simulink model "VIPL4sStEnCtrl"  (R2018b)
settings: Solver=FixedStepDiscrete  StartTime=0.0  StopTime=10.0  FixedStep=0.01  RelTol=1e-3
undefined symbols (not defined in the file or in its folder): data, KeSMSw4SSecRwLtStLgrstUpwdDnwdOpenPos1_Val, SecRwLtStBkReclnEn_Clear, SecRwLtStBkReclnEn_Set, SecRwLtStFtrstEn_Clear, SecRwLtStFtrstEn_Set, SecRwLtStFwdBkwdEn_Clear, SecRwLtStFwdBkwdEn_Set, SecRwLtStHdrstFwdBkwdEn_Clear, SecRwLtStHdrstFwdBkwdEn_Set, SecRwLtStHdrstUpwdDnwdEn_Clear, SecRwLtStHdrstUpwdDnwdEn_Set, SecRwLtStLgrstInwdOtwdEn_Clear, SecRwLtStLgrstInwdOtwdEn_Set, SecRwLtStLgrstUpwdDnwdEn_Clear, SecRwLtStLgrstUpwdDnwdEn_Set
libraries: simulink x16
settings Model: ModifiedHistory="2023.11.16  V2.3.0 Issue 566045 全躺，vip，腿托打开增加前后位置"  Creator=sn2xws  LastModifiedBy=sn2xws
settings DataIOCC: SaveFormat=StructureWithTime
settings OptimizationCC: DefaultParameterBehavior=Inlined  EnhancedBackFolding=on  PassReuseOutputArgsAs=Individual arguments  ZeroExternalMemoryAtStartup=off  ZeroInternalMemoryAtStartup=off  OptimizeBlockOrder=speed  DifferentSizesBufferReuse=on  OptimizationCustomize=off
settings DebuggingCC: ParameterTunabilityLossMsg=error
settings SFSimCC: MATLABDynamicMemAlloc=off
settings RTWCC: SystemTargetFile=autosar.tlc  GenCodeOnly=on  TemplateMakefile=ert_default_tmf  Description=AUTOSAR  GenerateReport=on  IncludeHyperlinkInReport=on  LaunchReport=on  GenerateTraceInfo=on  GenerateTraceReport=on  GenerateTraceReportSl=on  GenerateTraceReportSf=on  GenerateTraceReportEml=on  GenerateCodeMetricsReport=on
settings CodeAppCC: ForceParamTrailComments=on  IgnoreCustomStorageClasses=off  OperatorAnnotations=on  SimulinkDataObjDesc=on  SFDataObjDesc=on  InsertBlockDesc=on
settings STFCustomTargetCC: TargetLangStandard=C99 (ISO)  MultiwordLength=256  ParMdlRefBuildCompliant=on  CompOptLevelCompliant=on  IncludeMdlTerminateFcn=off  CombineOutputUpdateFcns=on  SuppressErrorStatus=on  ERTCustomFileBanners=on  SupportNonFinite=off  SupportComplex=off  SupportContinuousTime=off  SupportNonInlinedSFcns=off  RemoveResetFunc=on  MATLABClassNameForMDSCustomization=Simulink.SoftwareTarget.ERTCustomization  AutosarCompliant=on  UseToolchainInfoCompliant=on  LookupTableObjectStructAxisOrder=2,1,3,4,...  LUTObjectStructOrderEvenSpacing=Size,Table,Breakpoints  SystemTargetFile=autosar.tlc
settings ERTTargetCC: TargetLangStandard=C99 (ISO)  ConcurrentExecutionCompliant=off  IncludeMdlTerminateFcn=off  SuppressErrorStatus=on  SupportNonFinite=off  SupportComplex=off  ModelStepFunctionPrototypeControlCompliant=off  CPPClassGenCompliant=off  AutosarCompliant=on  LookupTableObjectStructAxisOrder=2,1,3,4,...  LUTObjectStructOrderEvenSpacing=Size,Table,Breakpoints  InlinedParameterPlacement=NonHierarchical  ERTCustomFileTemplate=example_file_process.tlc  ERTFilePackagingFormat=Compact

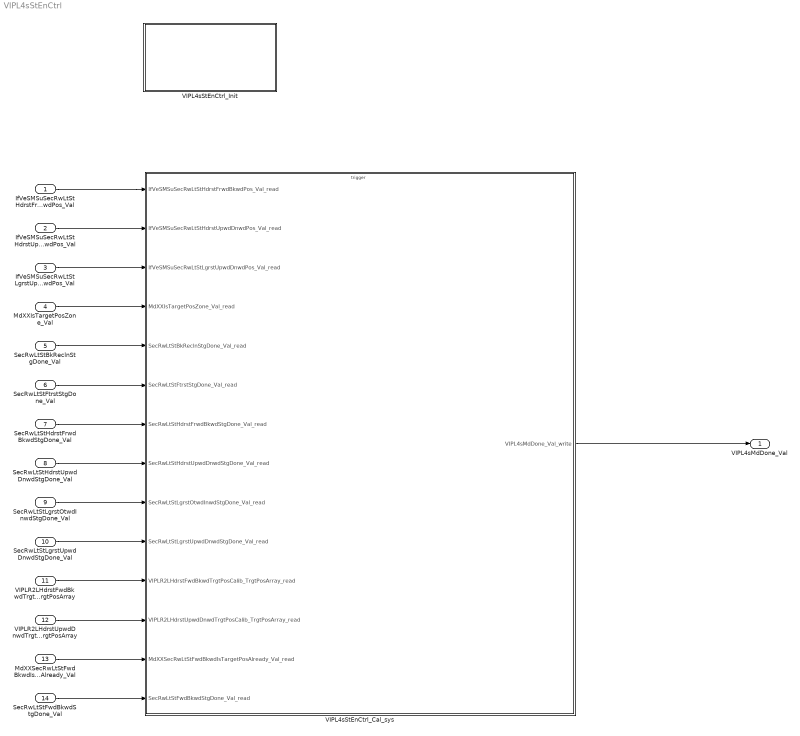
== system VIPL4sStEnCtrl ==
  IfVeSMSuSecRwLtStHdrstFrwdBkwdPos_Val : Inport  OutDataTypeStr=uint16  PortDimensions=1
  IfVeSMSuSecRwLtStHdrstUpwdDnwdPos_Val : Inport  Port=2  OutDataTypeStr=uint16  PortDimensions=1
  IfVeSMSuSecRwLtStLgrstUpwdDnwdPos_Val : Inport  Port=3  OutDataTypeStr=uint16  PortDimensions=1
  MdXXIsTargetPosZone_Val : Inport  Port=4  OutDataTypeStr=uint32  PortDimensions=1
  SecRwLtStBkReclnStgDone_Val : Inport  Port=5  OutDataTypeStr=boolean  PortDimensions=1
  SecRwLtStFtrstStgDone_Val : Inport  Port=6  OutDataTypeStr=boolean  PortDimensions=1
  SecRwLtStHdrstFrwdBkwdStgDone_Val : Inport  Port=7  OutDataTypeStr=boolean  PortDimensions=1
  SecRwLtStHdrstUpwdDnwdStgDone_Val : Inport  Port=8  OutDataTypeStr=boolean  PortDimensions=1
  SecRwLtStLgrstOtwdInwdStgDone_Val : Inport  Port=9  OutDataTypeStr=boolean  PortDimensions=1
  SecRwLtStLgrstUpwdDnwdStgDone_Val : Inport  Port=10  OutDataTypeStr=boolean  PortDimensions=1
  VIPLR2LHdrstFwdBkwdTrgtPosCalib_TrgtPosArray : Inport  Description=|  Port=11  OutDataTypeStr=uint16  PortDimensions=3
      | 0:Pos
      | 1:Max
      | 2:Min
  VIPLR2LHdrstUpwdDnwdTrgtPosCalib_TrgtPosArray : Inport  Description=|  Port=12  OutDataTypeStr=uint16  PortDimensions=3
      | 0:Pos
      | 1:Max
      | 2:Min
  MdXXSecRwLtStFwdBkwdIsTargetPosAlready_Val : Inport  Port=13  OutDataTypeStr=uint32  PortDimensions=1
  SecRwLtStFwdBkwdStgDone_Val : Inport  Port=14  OutDataTypeStr=boolean  PortDimensions=1
  VIPL4sStEnCtrl_Cal_sys : Subsystem
  VIPL4sStEnCtrl_Init : Subsystem
  VIPL4sMdDone_Val : Outport  OutDataTypeStr=uint8  PortDimensions=1
  wires:
  IfVeSMSuSecRwLtStHdrstFrwdBkwdPos_Val/1 -> VIPL4sStEnCtrl_Cal_sys/1(IfVeSMSuSecRwLtStHdrstFrwdBkwdPos_Val_read)
  IfVeSMSuSecRwLtStHdrstUpwdDnwdPos_Val/1 -> VIPL4sStEnCtrl_Cal_sys/2(IfVeSMSuSecRwLtStHdrstUpwdDnwdPos_Val_read)
  IfVeSMSuSecRwLtStLgrstUpwdDnwdPos_Val/1 -> VIPL4sStEnCtrl_Cal_sys/3(IfVeSMSuSecRwLtStLgrstUpwdDnwdPos_Val_read)
  MdXXIsTargetPosZone_Val/1 -> VIPL4sStEnCtrl_Cal_sys/4(MdXXIsTargetPosZone_Val_read)
  SecRwLtStBkReclnStgDone_Val/1 -> VIPL4sStEnCtrl_Cal_sys/5(SecRwLtStBkReclnStgDone_Val_read)
  SecRwLtStFtrstStgDone_Val/1 -> VIPL4sStEnCtrl_Cal_sys/6(SecRwLtStFtrstStgDone_Val_read)
  SecRwLtStHdrstFrwdBkwdStgDone_Val/1 -> VIPL4sStEnCtrl_Cal_sys/7(SecRwLtStHdrstFrwdBkwdStgDone_Val_read)
  SecRwLtStHdrstUpwdDnwdStgDone_Val/1 -> VIPL4sStEnCtrl_Cal_sys/8(SecRwLtStHdrstUpwdDnwdStgDone_Val_read)
  SecRwLtStLgrstOtwdInwdStgDone_Val/1 -> VIPL4sStEnCtrl_Cal_sys/9(SecRwLtStLgrstOtwdInwdStgDone_Val_read)
  SecRwLtStLgrstUpwdDnwdStgDone_Val/1 -> VIPL4sStEnCtrl_Cal_sys/10(SecRwLtStLgrstUpwdDnwdStgDone_Val_read)
  VIPLR2LHdrstFwdBkwdTrgtPosCalib_TrgtPosArray/1 -> VIPL4sStEnCtrl_Cal_sys/11(VIPLR2LHdrstFwdBkwdTrgtPosCalib_TrgtPosArray_read)
  VIPLR2LHdrstUpwdDnwdTrgtPosCalib_TrgtPosArray/1 -> VIPL4sStEnCtrl_Cal_sys/12(VIPLR2LHdrstUpwdDnwdTrgtPosCalib_TrgtPosArray_read)
  VIPL4sStEnCtrl_Cal_sys/1(VIPL4sMdDone_Val_write) -> VIPL4sMdDone_Val/1
  MdXXSecRwLtStFwdBkwdIsTargetPosAlready_Val/1 -> VIPL4sStEnCtrl_Cal_sys/13(MdXXSecRwLtStFwdBkwdIsTargetPosAlready_Val_read)
  SecRwLtStFwdBkwdStgDone_Val/1 -> VIPL4sStEnCtrl_Cal_sys/14(SecRwLtStFwdBkwdStgDone_Val_read)

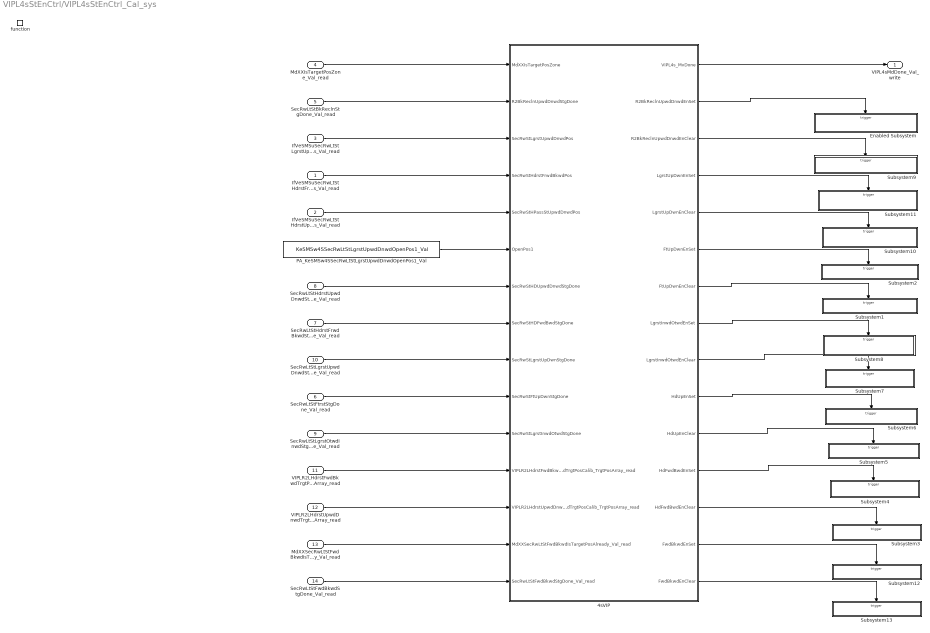
== system VIPL4sStEnCtrl/VIPL4sStEnCtrl_Cal_sys ==
  IfVeSMSuSecRwLtStHdrstFrwdBkwdPos_Val_read : Inport
  IfVeSMSuSecRwLtStHdrstUpwdDnwdPos_Val_read : Inport  Port=2
  IfVeSMSuSecRwLtStLgrstUpwdDnwdPos_Val_read : Inport  Port=3
  MdXXIsTargetPosZone_Val_read : Inport  Port=4
  SecRwLtStBkReclnStgDone_Val_read : Inport  Port=5
  SecRwLtStFtrstStgDone_Val_read : Inport  Port=6
  SecRwLtStHdrstFrwdBkwdStgDone_Val_read : Inport  Port=7
  SecRwLtStHdrstUpwdDnwdStgDone_Val_read : Inport  Port=8
  SecRwLtStLgrstOtwdInwdStgDone_Val_read : Inport  Port=9
  SecRwLtStLgrstUpwdDnwdStgDone_Val_read : Inport  Port=10
  VIPLR2LHdrstFwdBkwdTrgtPosCalib_TrgtPosArray_read : Inport  Port=11
  VIPLR2LHdrstUpwdDnwdTrgtPosCalib_TrgtPosArray_read : Inport  Port=12
  MdXXSecRwLtStFwdBkwdIsTargetPosAlready_Val_read : Inport  Port=13
  SecRwLtStFwdBkwdStgDone_Val_read : Inport  Port=14
  function : TriggerPort  TriggerType=function-call  IsSimulinkFunction=on  FunctionName=VIPL4sStEnCtrl_Cal  VariantControl=(inherit)
  4sVIP : Subsystem
  Enabled Subsystem : Subsystem  TreatAsAtomicUnit=on
  PA_KeSMSw4SSecRwLtStLgrstUpwdDnwdOpenPos1_Val : Constant  Value=KeSMSw4SSecRwLtStLgrstUpwdDnwdOpenPos1_Val
  Subsystem1 : Subsystem
  Subsystem10 : Subsystem
  Subsystem11 : Subsystem
  Subsystem12 : Subsystem
  Subsystem13 : Subsystem
  Subsystem2 : Subsystem
  Subsystem3 : Subsystem
  Subsystem4 : Subsystem
  Subsystem5 : Subsystem
  Subsystem6 : Subsystem
  Subsystem7 : Subsystem
  Subsystem8 : Subsystem
  Subsystem9 : Subsystem
  VIPL4sMdDone_Val_write : Outport
      settings: EnsureOutportIsVirtual=on
  wires:
  4sVIP/1(VIPL4s_MvDone) -> VIPL4sMdDone_Val_write/1
  PA_KeSMSw4SSecRwLtStLgrstUpwdDnwdOpenPos1_Val/1 -> 4sVIP/6(OpenPos1)
  MdXXIsTargetPosZone_Val_read/1 -> 4sVIP/1(MdXXIsTargetPosZone)
  SecRwLtStBkReclnStgDone_Val_read/1 -> 4sVIP/2(R2BkReclnUpwdDnwdStgDone)
  IfVeSMSuSecRwLtStLgrstUpwdDnwdPos_Val_read/1 -> 4sVIP/3(SecRwStLgrstUpwdDnwdPos)
  IfVeSMSuSecRwLtStHdrstFrwdBkwdPos_Val_read/1 -> 4sVIP/4(SecRwStHdrstFrwdBkwdPos)
  IfVeSMSuSecRwLtStHdrstUpwdDnwdPos_Val_read/1 -> 4sVIP/5(SecRwStHPassStUpwdDnwdPos)
  SecRwLtStFtrstStgDone_Val_read/1 -> 4sVIP/10(SecRwStFtUpDwnStgDone)
  SecRwLtStLgrstOtwdInwdStgDone_Val_read/1 -> 4sVIP/11(SecRwStLgrstInwdOtwdStgDone)
  SecRwLtStLgrstUpwdDnwdStgDone_Val_read/1 -> 4sVIP/9(SecRwStLgrstUpDwnStgDone)
  SecRwLtStHdrstFrwdBkwdStgDone_Val_read/1 -> 4sVIP/8(SecRwStHDFwdBwdStgDone)
  SecRwLtStHdrstUpwdDnwdStgDone_Val_read/1 -> 4sVIP/7(SecRwStHDUpwdDnwdStgDone)
  VIPLR2LHdrstFwdBkwdTrgtPosCalib_TrgtPosArray_read/1 -> 4sVIP/12(VIPLR2LHdrstFwdBkwdTrgtPosCalib_TrgtPosArray_read)
  VIPLR2LHdrstUpwdDnwdTrgtPosCalib_TrgtPosArray_read/1 -> 4sVIP/13(VIPLR2LHdrstUpwdDnwdTrgtPosCalib_TrgtPosArray_read)
  4sVIP/3(R2BkReclnUpwdDnwdEnClear) -> Subsystem9/Trigger
  4sVIP/12(HdFwdBwdEnSet) -> Subsystem4/Trigger
  4sVIP/6(FtUpDwnEnSet) -> Subsystem2/Trigger
  4sVIP/11(HdUpEnClear) -> Subsystem5/Trigger
  4sVIP/7(FtUpDwnEnClear) -> Subsystem1/Trigger
  4sVIP/13(HdFwdBwdEnClear) -> Subsystem3/Trigger
  4sVIP/2(R2BkReclnUpwdDnwdEnSet) -> Enabled Subsystem/Trigger
  4sVIP/10(HdUpEnSet) -> Subsystem6/Trigger
  4sVIP/4(LgrstUpDwnEnSet) -> Subsystem11/Trigger
  4sVIP/9(LgrstInwdOtwdEnClear) -> Subsystem7/Trigger
  4sVIP/8(LgrstInwdOtwdEnSet) -> Subsystem8/Trigger
  4sVIP/5(LgrstUpDwnEnClear) -> Subsystem10/Trigger
  MdXXSecRwLtStFwdBkwdIsTargetPosAlready_Val_read/1 -> 4sVIP/14(MdXXSecRwLtStFwdBkwdIsTargetPosAlready_Val_read)
  SecRwLtStFwdBkwdStgDone_Val_read/1 -> 4sVIP/15(SecRwLtStFwdBkwdStgDone_Val_read)
  4sVIP/14(FwdBkwdEnSet) -> Subsystem12/Trigger
  4sVIP/15(FwdBkwdEnClear) -> Subsystem13/Trigger

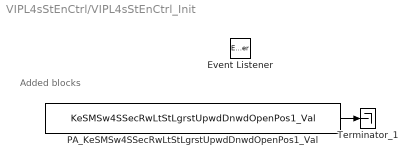
== system VIPL4sStEnCtrl/VIPL4sStEnCtrl_Init ==
  note: Added blocks
  Event Listener : EventListener  EventName=reset
  PA_KeSMSw4SSecRwLtStLgrstUpwdDnwdOpenPos1_Val : Constant  Value=KeSMSw4SSecRwLtStLgrstUpwdDnwdOpenPos1_Val
  Terminator_1 : Terminator
  wires:
  PA_KeSMSw4SSecRwLtStLgrstUpwdDnwdOpenPos1_Val/1 -> Terminator_1/1

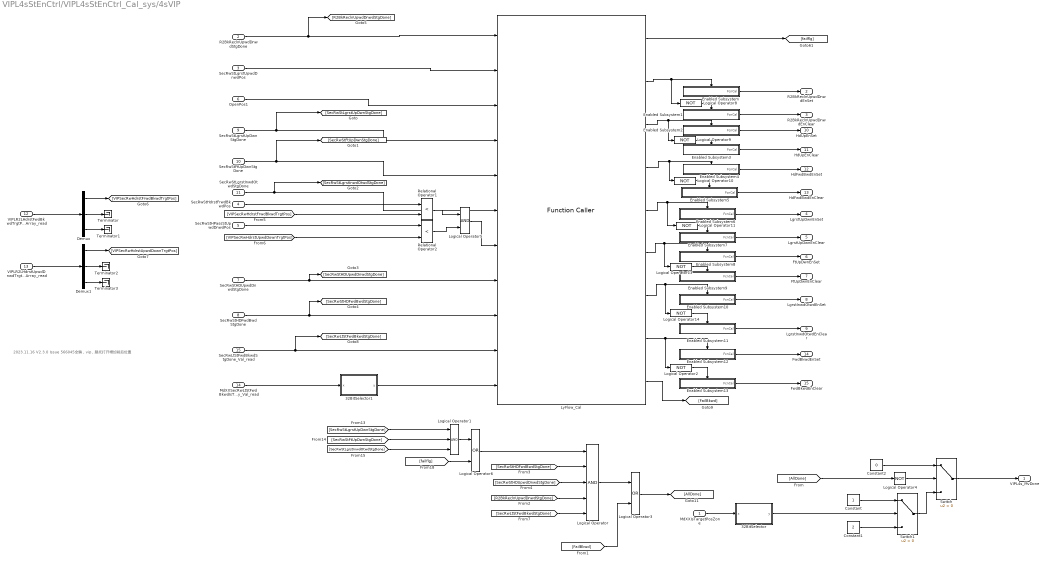
== system VIPL4sStEnCtrl/VIPL4sStEnCtrl_Cal_sys/4sVIP ==
  note: 2023.11.16 V2.3.0 Issue 566045 全躺，vip，腿托打开增加前后位置
  MdXXIsTargetPosZone : Inport
  R2BkReclnUpwdDnwdStgDone : Inport  Port=2
  SecRwStLgrstUpwdDnwdPos : Inport  Port=3
  SecRwStHdrstFrwdBkwdPos : Inport  Port=4
  SecRwStHPassStUpwdDnwdPos : Inport  Port=5
  OpenPos1 : Inport  Port=6
  SecRwStHDUpwdDnwdStgDone : Inport  Port=7
  SecRwStHDFwdBwdStgDone : Inport  Port=8
  SecRwStLgrstUpDwnStgDone : Inport  Port=9
  SecRwStFtUpDwnStgDone : Inport  Port=10
  SecRwStLgrstInwdOtwdStgDone : Inport  Port=11
  VIPLR2LHdrstFwdBkwdTrgtPosCalib_TrgtPosArray_read : Inport  Port=12
  VIPLR2LHdrstUpwdDnwdTrgtPosCalib_TrgtPosArray_read : Inport  Port=13
  MdXXSecRwLtStFwdBkwdIsTargetPosAlready_Val_read : Inport  Port=14
  SecRwLtStFwdBkwdStgDone_Val_read : Inport  Port=15
  32BitSelector : Subsystem  mask(32 Bit Selector){BitNum=9}
      mask prompts: BitNum "Select Bit Number"
      mask help: Allows selection of a particular bit (0-31) out of a packed word up to 32 bits long. Output will be true if the bit number selected via the mask parameter is equal to one.
      mask TypeOptions BitNum: 0 | 1 | 2 | 3 | 4 | 5 | 6 | 7 | 8 | 9 | 10 | 11 | 12 | 13 | 14 | 15 | 16 | 17 | 18 | 19 | 20 | 21 | 22 | 23 | 24 | 25 | 26 | 27 | 28 | 29 | 30 | 31
      mask Display:
      | text(0.5, 0.8,'BIT','horizontalAlignment','center')
      | text(0.5, 0.5,'SELECTOR','horizontalAlignment','center')
      | text(0.5, 0.2,['-- Bit ',char(get_param(gcb,'BitNum')),' --'],'horizontalAlignment','center')
  32BitSelector1 : Subsystem  mask(32 Bit Selector){BitNum=9}
      mask prompts: BitNum "Select Bit Number"
      mask help: Allows selection of a particular bit (0-31) out of a packed word up to 32 bits long. Output will be true if the bit number selected via the mask parameter is equal to one.
      mask TypeOptions BitNum: 0 | 1 | 2 | 3 | 4 | 5 | 6 | 7 | 8 | 9 | 10 | 11 | 12 | 13 | 14 | 15 | 16 | 17 | 18 | 19 | 20 | 21 | 22 | 23 | 24 | 25 | 26 | 27 | 28 | 29 | 30 | 31
      mask Display:
      | text(0.5, 0.8,'BIT','horizontalAlignment','center')
      | text(0.5, 0.5,'SELECTOR','horizontalAlignment','center')
      | text(0.5, 0.2,['-- Bit ',char(get_param(gcb,'BitNum')),' --'],'horizontalAlignment','center')
  Constant : Constant  OutDataTypeStr=uint8
  Constant1 : Constant  Value=2  OutDataTypeStr=uint8
  Constant2 : Constant  Value=0  OutDataTypeStr=uint8
  Demux : Demux  Outputs=3
  Demux1 : Demux  Outputs=3
  Enabled Subsystem : Subsystem  TreatAsAtomicUnit=on
  Enabled Subsystem1 : Subsystem  TreatAsAtomicUnit=on
  Enabled Subsystem10 : Subsystem  TreatAsAtomicUnit=on
  Enabled Subsystem11 : Subsystem  TreatAsAtomicUnit=on
  Enabled Subsystem12 : Subsystem  TreatAsAtomicUnit=on
  Enabled Subsystem13 : Subsystem  TreatAsAtomicUnit=on
  Enabled Subsystem2 : Subsystem  TreatAsAtomicUnit=on
  Enabled Subsystem3 : Subsystem  TreatAsAtomicUnit=on
  Enabled Subsystem4 : Subsystem  TreatAsAtomicUnit=on
  Enabled Subsystem5 : Subsystem  TreatAsAtomicUnit=on
  Enabled Subsystem6 : Subsystem  TreatAsAtomicUnit=on
  Enabled Subsystem7 : Subsystem  TreatAsAtomicUnit=on
  Enabled Subsystem8 : Subsystem  TreatAsAtomicUnit=on
  Enabled Subsystem9 : Subsystem  TreatAsAtomicUnit=on
  Logical Operator : Logic  Inputs=5  AllPortsSameDT=off  OutDataTypeStr=boolean
  Logical Operator1 : Logic  Inputs=3  AllPortsSameDT=off  OutDataTypeStr=boolean
  Logical Operator{2,4,8..11,13..14} (8 alike) : Logic  Operator=NOT  AllPortsSameDT=off  OutDataTypeStr=boolean
  Logical Operator3 : Logic  Operator=OR  AllPortsSameDT=off  OutDataTypeStr=boolean
  Logical Operator5 : Logic  AllPortsSameDT=off  OutDataTypeStr=boolean
  Logical Operator6 : Logic  Operator=OR  AllPortsSameDT=off  OutDataTypeStr=boolean
  LyFlow_Cal : FunctionCaller  FunctionPrototype=[Failflg,BkReclnEn,HdrstUpwdEn,HdrstFrwdEn,LgrstUpwdDnwdEn,FtrstEn,LgrstInwdOtwdEn,FwdBkwdEn,FailBkwd] = LyFlow_Cal(BkReclnStgDone,LgrstUpwdDnwdPos,LgrstUpwdDnwdOpenPos1,LgrstUpwdStgDone,FtrstStgDone,LgrstInwdStgDone,Chkhdflg,HdrstUpwdDnwdStgDone,HdrstFrwdBkwdStgDone,FwdBkwdStgDone,FwdBkwdIsPosAlready)  InputArgumentSpecifications=boolean(true), uint16(1), uint16(1), boolean(true), boolean(true), boolean(true), boolean(true), boolean(true), boolean(true), boolean(true), boolean(true)  OutputArgumentSpecifications=boolean(true), boolean(true), boolean(true), boolean(true), boolean(true), boolean(true), boolean(true), boolean(true), boolean(true)
  Relational Operator1 : RelationalOperator  Operator=<  OutDataTypeStr=boolean  RndMeth=Simplest
  Relational Operator2 : RelationalOperator  Operator=<  OutDataTypeStr=boolean  RndMeth=Simplest
  Switch : Switch  Criteria=u2 > Threshold
  Switch1 : Switch  Criteria=u2 > Threshold
  Terminator{,1..3} (4 alike) : Terminator
  VIPL4s_MvDone : Outport
  R2BkReclnUpwdDnwdEnSet : Outport  Port=2
  R2BkReclnUpwdDnwdEnClear : Outport  Port=3
  LgrstUpDwnEnSet : Outport  Port=4
  LgrstUpDwnEnClear : Outport  Port=5
  FtUpDwnEnSet : Outport  Port=6
  FtUpDwnEnClear : Outport  Port=7
  LgrstInwdOtwdEnSet : Outport  Port=8
  LgrstInwdOtwdEnClear : Outport  Port=9
  HdUpEnSet : Outport  Port=10
  HdUpEnClear : Outport  Port=11
  HdFwdBwdEnSet : Outport  Port=12
  HdFwdBwdEnClear : Outport  Port=13
  FwdBkwdEnSet : Outport  Port=14
  FwdBkwdEnClear : Outport  Port=15
  wires:
  [VIPSecRwHdrstUpwdDownTrgtPos] -> Relational Operator2/2
  [R2BkReclnUpwdDnwdStgDone] -> Logical Operator/4
  [SecRwStFtUpDwnStgDone] -> Logical Operator1/2
  [SecRwStHDFwdBwdStgDone] -> Logical Operator/2
  SecRwStHDFwdBwdStgDone/1 -> [SecRwStHDFwdBwdStgDone], LyFlow_Cal/9
  Logical Operator5/1 -> LyFlow_Cal/7
  OpenPos1/1 -> LyFlow_Cal/3
  SecRwStLgrstInwdOtwdStgDone/1 -> [SecRwStLgrstInwdOtwdStgDone], LyFlow_Cal/6
  [failflg] -> Logical Operator6/2
  SecRwStHdrstFrwdBkwdPos/1 -> Relational Operator1/1
  Relational Operator2/1 -> Logical Operator5/2
  SecRwStFtUpDwnStgDone/1 -> [SecRwStFtUpDwnStgDone], LyFlow_Cal/5
  [SecRwStLgrstInwdOtwdStgDone] -> Logical Operator1/3
  SecRwStHPassStUpwdDnwdPos/1 -> Relational Operator2/1
  [SecRwStLgrstUpDwnStgDone] -> Logical Operator1/1
  Logical Operator1/1 -> Logical Operator6/1
  Logical Operator6/1 -> Logical Operator/1
  [SecRwStHDUpwdDnwdStgDone] -> Logical Operator/3
  MdXXIsTargetPosZone/1 -> 32BitSelector/1(x)
  Relational Operator1/1 -> Logical Operator5/1
  SecRwStHDUpwdDnwdStgDone/1 -> [SecRwStHDUpwdDnwdStgDone], LyFlow_Cal/8
  LyFlow_Cal/1 -> [failflg]
  SecRwStLgrstUpwdDnwdPos/1 -> LyFlow_Cal/2
  R2BkReclnUpwdDnwdStgDone/1 -> [R2BkReclnUpwdDnwdStgDone], LyFlow_Cal/1
  [VIPSecRwHdrstFrwdBkwdTrgtPos] -> Relational Operator1/2
  SecRwStLgrstUpDwnStgDone/1 -> [SecRwStLgrstUpDwnStgDone], LyFlow_Cal/4
  Switch/1 -> VIPL4s_MvDone/1
  Switch1/1 -> Switch/3
  LyFlow_Cal/6 -> Logical Operator13/1, Enabled Subsystem8/Enable
  Enabled Subsystem1/1(FcnCal) -> R2BkReclnUpwdDnwdEnClear/1
  Enabled Subsystem6/1(FcnCal) -> LgrstUpDwnEnSet/1
  Enabled Subsystem9/1(FcnCal) -> FtUpDwnEnClear/1
  Enabled Subsystem8/1(FcnCal) -> FtUpDwnEnSet/1
  Enabled Subsystem11/1(FcnCal) -> LgrstInwdOtwdEnClear/1
  Enabled Subsystem7/1(FcnCal) -> LgrstUpDwnEnClear/1
  LyFlow_Cal/7 -> Logical Operator14/1, Enabled Subsystem10/Enable
  Enabled Subsystem5/1(FcnCal) -> HdFwdBwdEnClear/1
  Logical Operator9/1 -> Enabled Subsystem3/Enable
  Enabled Subsystem2/1(FcnCal) -> HdUpEnSet/1
  LyFlow_Cal/5 -> Logical Operator11/1, Enabled Subsystem6/Enable
  Enabled Subsystem4/1(FcnCal) -> HdFwdBwdEnSet/1
  Enabled Subsystem/1(FcnCal) -> R2BkReclnUpwdDnwdEnSet/1
  Enabled Subsystem10/1(FcnCal) -> LgrstInwdOtwdEnSet/1
  Enabled Subsystem3/1(FcnCal) -> HdUpEnClear/1
  Logical Operator8/1 -> Enabled Subsystem1/Enable
  LyFlow_Cal/3 -> Logical Operator9/1, Enabled Subsystem2/Enable
  Logical Operator13/1 -> Enabled Subsystem9/Enable
  Logical Operator14/1 -> Enabled Subsystem11/Enable
  LyFlow_Cal/4 -> Logical Operator10/1, Enabled Subsystem4/Enable
  Logical Operator11/1 -> Enabled Subsystem7/Enable
  Logical Operator10/1 -> Enabled Subsystem5/Enable
  LyFlow_Cal/2 -> Logical Operator8/1, Enabled Subsystem/Enable
  VIPLR2LHdrstFwdBkwdTrgtPosCalib_TrgtPosArray_read/1 -> Demux/1
  Demux/1 -> [VIPSecRwHdrstFrwdBkwdTrgtPos]
  Demux/2 -> Terminator/1
  Demux/3 -> Terminator1/1
  VIPLR2LHdrstUpwdDnwdTrgtPosCalib_TrgtPosArray_read/1 -> Demux1/1
  Demux1/1 -> [VIPSecRwHdrstUpwdDownTrgtPos]
  Demux1/2 -> Terminator2/1
  Demux1/3 -> Terminator3/1
  Constant2/1 -> Switch/1
  Constant1/1 -> Switch1/3
  Constant/1 -> Switch1/1
  [AllDone] -> Logical Operator4/1
  Logical Operator4/1 -> Switch/2
  32BitSelector/1(y) -> Switch1/2
  SecRwLtStFwdBkwdStgDone_Val_read/1 -> [SecRwLtStFwdBkwdStgDone], LyFlow_Cal/10
  MdXXSecRwLtStFwdBkwdIsTargetPosAlready_Val_read/1 -> 32BitSelector1/1(x)
  Logical Operator2/1 -> Enabled Subsystem13/Enable
  Enabled Subsystem12/1(FcnCal) -> FwdBkwdEnSet/1
  LyFlow_Cal/8 -> Enabled Subsystem12/Enable, Logical Operator2/1
  Enabled Subsystem13/1(FcnCal) -> FwdBkwdEnClear/1
  LyFlow_Cal/9 -> [FailBkwd]
  Logical Operator/1 -> Logical Operator3/1
  [FailBkwd] -> Logical Operator3/2
  Logical Operator3/1 -> [AllDone]
  [SecRwLtStFwdBkwdStgDone] -> Logical Operator/5
  32BitSelector1/1(y) -> LyFlow_Cal/11

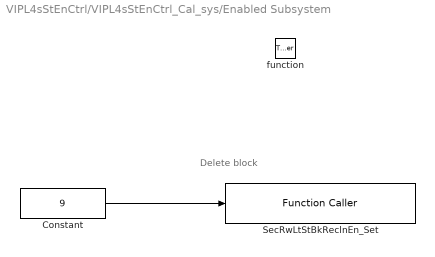
== system VIPL4sStEnCtrl/VIPL4sStEnCtrl_Cal_sys/Enabled Subsystem ==
  note: Delete block
  function : TriggerPort  TriggerType=function-call  VariantControl=Variant
  Constant : Constant  Value=9  OutDataTypeStr=uint8
  SecRwLtStBkReclnEn_Set : FunctionCaller  FunctionPrototype=SecRwLtStBkReclnEn_Set(data)  InputArgumentSpecifications=uint8(1)
  wires:
  Constant/1 -> SecRwLtStBkReclnEn_Set/1

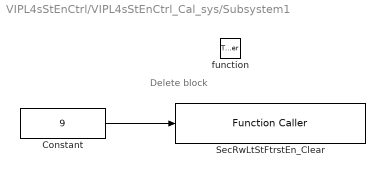
== system VIPL4sStEnCtrl/VIPL4sStEnCtrl_Cal_sys/Subsystem1 ==
  note: Delete block
  function : TriggerPort  TriggerType=function-call  VariantControl=Variant
  Constant : Constant  Value=9  OutDataTypeStr=uint8
  SecRwLtStFtrstEn_Clear : FunctionCaller  FunctionPrototype=SecRwLtStFtrstEn_Clear(data)  InputArgumentSpecifications=uint8(1)
  wires:
  Constant/1 -> SecRwLtStFtrstEn_Clear/1

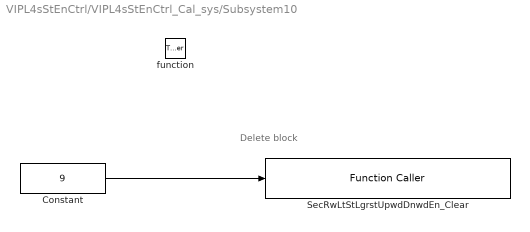
== system VIPL4sStEnCtrl/VIPL4sStEnCtrl_Cal_sys/Subsystem10 ==
  note: Delete block
  function : TriggerPort  TriggerType=function-call  VariantControl=Variant
  Constant : Constant  Value=9  OutDataTypeStr=uint8
  SecRwLtStLgrstUpwdDnwdEn_Clear : FunctionCaller  FunctionPrototype=SecRwLtStLgrstUpwdDnwdEn_Clear(data)  InputArgumentSpecifications=uint8(1)
  wires:
  Constant/1 -> SecRwLtStLgrstUpwdDnwdEn_Clear/1

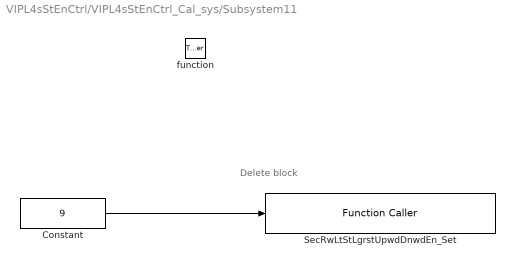
== system VIPL4sStEnCtrl/VIPL4sStEnCtrl_Cal_sys/Subsystem11 ==
  note: Delete block
  function : TriggerPort  TriggerType=function-call  VariantControl=Variant
  Constant : Constant  Value=9  OutDataTypeStr=uint8
  SecRwLtStLgrstUpwdDnwdEn_Set : FunctionCaller  FunctionPrototype=SecRwLtStLgrstUpwdDnwdEn_Set(data)  InputArgumentSpecifications=uint8(1)
  wires:
  Constant/1 -> SecRwLtStLgrstUpwdDnwdEn_Set/1

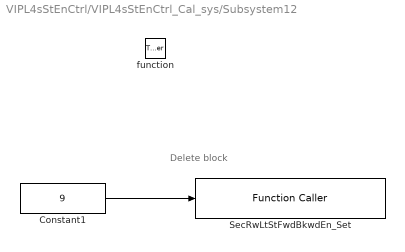
== system VIPL4sStEnCtrl/VIPL4sStEnCtrl_Cal_sys/Subsystem12 ==
  note: Delete block
  function : TriggerPort  TriggerType=function-call  VariantControl=Variant
  Constant1 : Constant  Value=9  OutDataTypeStr=uint8
  SecRwLtStFwdBkwdEn_Set : FunctionCaller  FunctionPrototype=SecRwLtStFwdBkwdEn_Set(data)  InputArgumentSpecifications=uint8(1)
  wires:
  Constant1/1 -> SecRwLtStFwdBkwdEn_Set/1

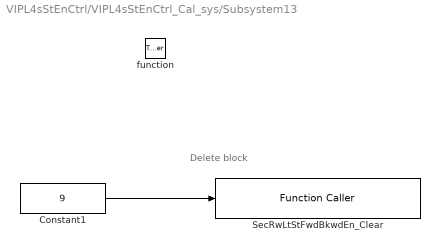
== system VIPL4sStEnCtrl/VIPL4sStEnCtrl_Cal_sys/Subsystem13 ==
  note: Delete block
  function : TriggerPort  TriggerType=function-call  VariantControl=Variant
  Constant1 : Constant  Value=9  OutDataTypeStr=uint8
  SecRwLtStFwdBkwdEn_Clear : FunctionCaller  FunctionPrototype=SecRwLtStFwdBkwdEn_Clear(data)  InputArgumentSpecifications=uint8(1)
  wires:
  Constant1/1 -> SecRwLtStFwdBkwdEn_Clear/1

== system VIPL4sStEnCtrl/VIPL4sStEnCtrl_Cal_sys/Subsystem2 ==
  note: Delete block
  function : TriggerPort  TriggerType=function-call  VariantControl=Variant
  Constant : Constant  Value=9  OutDataTypeStr=uint8
  SecRwLtStFtrstEn_Set : FunctionCaller  FunctionPrototype=SecRwLtStFtrstEn_Set(data)  InputArgumentSpecifications=uint8(1)
  wires:
  Constant/1 -> SecRwLtStFtrstEn_Set/1

== system VIPL4sStEnCtrl/VIPL4sStEnCtrl_Cal_sys/Subsystem3 ==
  note: Delete block
  function : TriggerPort  TriggerType=function-call  VariantControl=Variant
  Constant1 : Constant  Value=9  OutDataTypeStr=uint8
  SecRwLtStHdrstFwdBkwdEn_Clear : FunctionCaller  FunctionPrototype=SecRwLtStHdrstFwdBkwdEn_Clear(data)  InputArgumentSpecifications=uint8(1)
  wires:
  Constant1/1 -> SecRwLtStHdrstFwdBkwdEn_Clear/1

== system VIPL4sStEnCtrl/VIPL4sStEnCtrl_Cal_sys/Subsystem4 ==
  note: Delete block
  function : TriggerPort  TriggerType=function-call  VariantControl=Variant
  Constant2 : Constant  Value=9  OutDataTypeStr=uint8
  SecRwLtStHdrstFwdBkwdEn_Set : FunctionCaller  FunctionPrototype=SecRwLtStHdrstFwdBkwdEn_Set(data)  InputArgumentSpecifications=uint8(1)
  wires:
  Constant2/1 -> SecRwLtStHdrstFwdBkwdEn_Set/1

== system VIPL4sStEnCtrl/VIPL4sStEnCtrl_Cal_sys/Subsystem5 ==
  note: Delete block
  function : TriggerPort  TriggerType=function-call  VariantControl=Variant
  Constant3 : Constant  Value=9  OutDataTypeStr=uint8
  SecRwLtStHdrstUpwdDnwdEn_Clear : FunctionCaller  FunctionPrototype=SecRwLtStHdrstUpwdDnwdEn_Clear(data)  InputArgumentSpecifications=uint8(1)
  wires:
  Constant3/1 -> SecRwLtStHdrstUpwdDnwdEn_Clear/1

== system VIPL4sStEnCtrl/VIPL4sStEnCtrl_Cal_sys/Subsystem6 ==
  note: Delete block
  function : TriggerPort  TriggerType=function-call  VariantControl=Variant
  Constant4 : Constant  Value=9  OutDataTypeStr=uint8
  SecRwLtStHdrstUpwdDnwdEn_Set : FunctionCaller  FunctionPrototype=SecRwLtStHdrstUpwdDnwdEn_Set(data)  InputArgumentSpecifications=uint8(1)
  wires:
  Constant4/1 -> SecRwLtStHdrstUpwdDnwdEn_Set/1

== system VIPL4sStEnCtrl/VIPL4sStEnCtrl_Cal_sys/Subsystem7 ==
  note: Delete block
  function : TriggerPort  TriggerType=function-call  VariantControl=Variant
  Constant5 : Constant  Value=9  OutDataTypeStr=uint8
  SecRwLtStLgrstInwdOtwdEn_Clear : FunctionCaller  FunctionPrototype=SecRwLtStLgrstInwdOtwdEn_Clear(data)  InputArgumentSpecifications=uint8(1)
  wires:
  Constant5/1 -> SecRwLtStLgrstInwdOtwdEn_Clear/1

== system VIPL4sStEnCtrl/VIPL4sStEnCtrl_Cal_sys/Subsystem8 ==
  note: Delete block
  function : TriggerPort  TriggerType=function-call  VariantControl=Variant
  Constant6 : Constant  Value=9  OutDataTypeStr=uint8
  SecRwLtStLgrstInwdOtwdEn_Set : FunctionCaller  FunctionPrototype=SecRwLtStLgrstInwdOtwdEn_Set(data)  InputArgumentSpecifications=uint8(1)
  wires:
  Constant6/1 -> SecRwLtStLgrstInwdOtwdEn_Set/1

== system VIPL4sStEnCtrl/VIPL4sStEnCtrl_Cal_sys/Subsystem9 ==
  note: Delete block
  function : TriggerPort  TriggerType=function-call  VariantControl=Variant
  Constant1 : Constant  Value=9  OutDataTypeStr=uint8
  SecRwLtStBkReclnEn_Clear : FunctionCaller  FunctionPrototype=SecRwLtStBkReclnEn_Clear(data)  InputArgumentSpecifications=uint8(1)
  wires:
  Constant1/1 -> SecRwLtStBkReclnEn_Clear/1

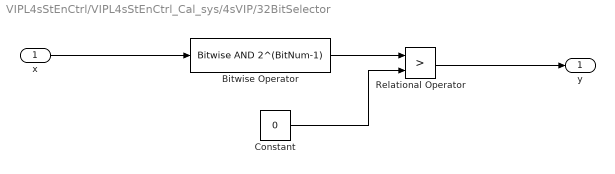
== system VIPL4sStEnCtrl/VIPL4sStEnCtrl_Cal_sys/4sVIP/32BitSelector ==
  x : Inport
  Bitwise Operator : simulink/Logic and Bit Operations/Bitwise Operator  logicop=AND  UseBitMask=on  BitMask=2^(BitNum-1)  BitMaskRealWorld=Stored Integer
  Constant : Constant  Value=0  OutDataTypeStr=uint32
  Relational Operator : RelationalOperator  Operator=>  OutDataTypeStr=boolean  RndMeth=Simplest
  y : Outport
  wires:
  Relational Operator/1 -> y/1
  Constant/1 -> Relational Operator/2
  x/1 -> Bitwise Operator/1
  Bitwise Operator/1 -> Relational Operator/1

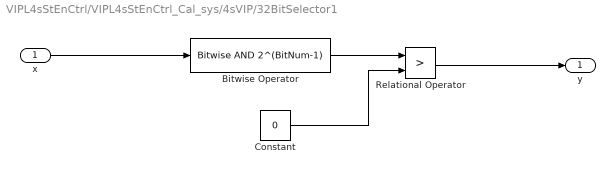
== system VIPL4sStEnCtrl/VIPL4sStEnCtrl_Cal_sys/4sVIP/32BitSelector1 ==
  x : Inport
  Bitwise Operator : simulink/Logic and Bit Operations/Bitwise Operator  logicop=AND  UseBitMask=on  BitMask=2^(BitNum-1)  BitMaskRealWorld=Stored Integer
  Constant : Constant  Value=0  OutDataTypeStr=uint32
  Relational Operator : RelationalOperator  Operator=>  OutDataTypeStr=boolean  RndMeth=Simplest
  y : Outport
  wires:
  Bitwise Operator/1 -> Relational Operator/1
  x/1 -> Bitwise Operator/1
  Constant/1 -> Relational Operator/2
  Relational Operator/1 -> y/1

== system VIPL4sStEnCtrl/VIPL4sStEnCtrl_Cal_sys/4sVIP/Enabled Subsystem ==
  Enable : EnablePort
  Function-Call Generator : simulink/Ports & Subsystems/Function-Call Generator  sample_time=-1  numberOfIterations=1
  FcnCal : Outport
  wires:
  Function-Call Generator/1 -> FcnCal/1

== system VIPL4sStEnCtrl/VIPL4sStEnCtrl_Cal_sys/4sVIP/Enabled Subsystem1 ==
  Enable : EnablePort
  Function-Call Generator : simulink/Ports & Subsystems/Function-Call Generator  sample_time=-1  numberOfIterations=1
  FcnCal : Outport
  wires:
  Function-Call Generator/1 -> FcnCal/1

== system VIPL4sStEnCtrl/VIPL4sStEnCtrl_Cal_sys/4sVIP/Enabled Subsystem10 ==
  Enable : EnablePort
  Function-Call Generator : simulink/Ports & Subsystems/Function-Call Generator  sample_time=-1  numberOfIterations=1
  FcnCal : Outport
  wires:
  Function-Call Generator/1 -> FcnCal/1

== system VIPL4sStEnCtrl/VIPL4sStEnCtrl_Cal_sys/4sVIP/Enabled Subsystem11 ==
  Enable : EnablePort
  Function-Call Generator : simulink/Ports & Subsystems/Function-Call Generator  sample_time=-1  numberOfIterations=1
  FcnCal : Outport
  wires:
  Function-Call Generator/1 -> FcnCal/1

== system VIPL4sStEnCtrl/VIPL4sStEnCtrl_Cal_sys/4sVIP/Enabled Subsystem12 ==
  Enable : EnablePort
  Function-Call Generator : simulink/Ports & Subsystems/Function-Call Generator  sample_time=-1  numberOfIterations=1
  FcnCal : Outport
  wires:
  Function-Call Generator/1 -> FcnCal/1

== system VIPL4sStEnCtrl/VIPL4sStEnCtrl_Cal_sys/4sVIP/Enabled Subsystem13 ==
  Enable : EnablePort
  Function-Call Generator : simulink/Ports & Subsystems/Function-Call Generator  sample_time=-1  numberOfIterations=1
  FcnCal : Outport
  wires:
  Function-Call Generator/1 -> FcnCal/1

== system VIPL4sStEnCtrl/VIPL4sStEnCtrl_Cal_sys/4sVIP/Enabled Subsystem2 ==
  Enable : EnablePort
  Function-Call Generator : simulink/Ports & Subsystems/Function-Call Generator  sample_time=-1  numberOfIterations=1
  FcnCal : Outport
  wires:
  Function-Call Generator/1 -> FcnCal/1

== system VIPL4sStEnCtrl/VIPL4sStEnCtrl_Cal_sys/4sVIP/Enabled Subsystem3 ==
  Enable : EnablePort
  Function-Call Generator : simulink/Ports & Subsystems/Function-Call Generator  sample_time=-1  numberOfIterations=1
  FcnCal : Outport
  wires:
  Function-Call Generator/1 -> FcnCal/1

== system VIPL4sStEnCtrl/VIPL4sStEnCtrl_Cal_sys/4sVIP/Enabled Subsystem4 ==
  Enable : EnablePort
  Function-Call Generator : simulink/Ports & Subsystems/Function-Call Generator  sample_time=-1  numberOfIterations=1
  FcnCal : Outport
  wires:
  Function-Call Generator/1 -> FcnCal/1

== system VIPL4sStEnCtrl/VIPL4sStEnCtrl_Cal_sys/4sVIP/Enabled Subsystem5 ==
  Enable : EnablePort
  Function-Call Generator : simulink/Ports & Subsystems/Function-Call Generator  sample_time=-1  numberOfIterations=1
  FcnCal : Outport
  wires:
  Function-Call Generator/1 -> FcnCal/1

== system VIPL4sStEnCtrl/VIPL4sStEnCtrl_Cal_sys/4sVIP/Enabled Subsystem6 ==
  Enable : EnablePort
  Function-Call Generator : simulink/Ports & Subsystems/Function-Call Generator  sample_time=-1  numberOfIterations=1
  FcnCal : Outport
  wires:
  Function-Call Generator/1 -> FcnCal/1

== system VIPL4sStEnCtrl/VIPL4sStEnCtrl_Cal_sys/4sVIP/Enabled Subsystem7 ==
  Enable : EnablePort
  Function-Call Generator : simulink/Ports & Subsystems/Function-Call Generator  sample_time=-1  numberOfIterations=1
  FcnCal : Outport
  wires:
  Function-Call Generator/1 -> FcnCal/1

== system VIPL4sStEnCtrl/VIPL4sStEnCtrl_Cal_sys/4sVIP/Enabled Subsystem8 ==
  Enable : EnablePort
  Function-Call Generator : simulink/Ports & Subsystems/Function-Call Generator  sample_time=-1  numberOfIterations=1
  FcnCal : Outport
  wires:
  Function-Call Generator/1 -> FcnCal/1

== system VIPL4sStEnCtrl/VIPL4sStEnCtrl_Cal_sys/4sVIP/Enabled Subsystem9 ==
  Enable : EnablePort
  Function-Call Generator : simulink/Ports & Subsystems/Function-Call Generator  sample_time=-1  numberOfIterations=1
  FcnCal : Outport
  wires:
  Function-Call Generator/1 -> FcnCal/1
